simulink model "feedforward"  (R2017a)
settings: Solver=VariableStepAuto  StartTime=0.0  StopTime=20  RelTol=1e-3
libraries: simulink x1
settings Model: Creator=faari  LastModifiedBy=faari

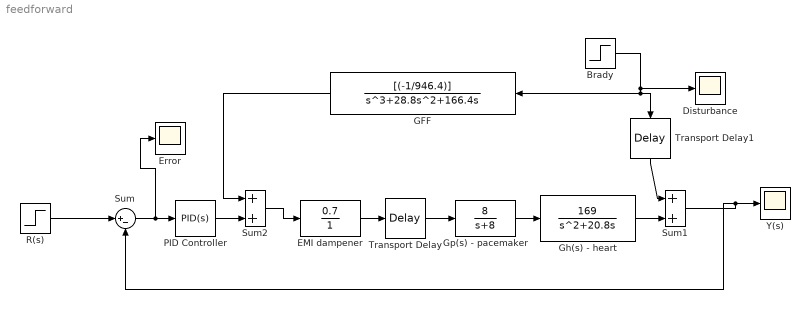
== system feedforward ==
  Brady : Step  Before=75  After=40  SampleTime=0
  Disturbance : Scope
  EMI dampener : TransferFcn  Numerator=[0.7]  Denominator=[1]
  Error : Scope
  GFF : TransferFcn  Numerator=[(-1/946.4)]  Denominator=[1 28.8 166.4 0]
  Gh(s) - heart : TransferFcn  Numerator=[169]  Denominator=[1 20.8 0]
  Gp(s) - pacemaker : TransferFcn  Numerator=[8]  Denominator=[1 8]
  PID Controller : simulink/Continuous/PID Controller  Controller=PID  TimeDomain=Continuous-time  SampleTime=-1  IntegratorMethod=Forward Euler  FilterMethod=Forward Euler  Form=Ideal  UseFilter=on  ControllerParametersSource=internal  P=0.475508627243744  I=0.245844606423706  D=0.157247274855767  N=100  InitialConditionSource=internal  InitialConditionForIntegrator=0  InitialConditionForFilter=0  ExternalReset=none  LimitOutput=off  UpperSaturationLimit=inf  LowerSaturationLimit=-inf  LinearizeAsGain=on  AntiWindupMode=none  Kb=1  TrackingMode=off  Kt=1  PParamMin=[]  PParamMax=[]  IParamMin=[]  IParamMax=[]  DParamMin=[]  DParamMax=[]  NParamMin=[]  NParamMax=[]  KbParamMin=[]  KbParamMax=[]  KtParamMin=[]  KtParamMax=[]  POutMin=[]  POutMax=[]  IOutMin=[]  IOutMax=[]  DOutMin=[]  DOutMax=[]  NOutMin=[]  NOutMax=[]  KbOutMin=[]  KbOutMax=[]  KtOutMin=[]  KtOutMax=[]  IntegratorOutMin=[]  IntegratorOutMax=[]  FilterOutMin=[]  FilterOutMax=[]  SumOutMin=[]  SumOutMax=[]  SumI1OutMin=[]  SumI1OutMax=[]  SumI2OutMin=[]  SumI2OutMax=[]  SumI3OutMin=[]  SumI3OutMax=[]  SumDOutMin=[]  SumDOutMax=[]  SaturationOutMin=[]  SaturationOutMax=[]  IntegratorContinuousStateAttributes=''  IntegratorStateMustResolveToSignalObject=off  IntegratorRTWStateStorageClass=Auto  FilterContinuousStateAttributes=''  FilterStateMustResolveToSignalObject=off  FilterRTWStateStorageClass=Auto  DifferentiatorICPrevScaledInput=0  DifferentiatorOutMin=[]  DifferentiatorOutMax=[]  InitialConditionSetting=State (most efficient)
  R(s) : Step  Time=0  After=75  SampleTime=0
  Sum : Sum  Inputs=|+-
  Sum1 : Sum  Inputs=+|+
  Sum2 : Sum  Inputs=+|+
  Transport Delay : TransportDelay  DelayTime=0.145
  Transport Delay1 : TransportDelay  DelayTime=0.145
  Y(s) : Scope
  wires:
  Sum/1 -> Error/1, PID Controller/1
  Gp(s) - pacemaker/1 -> Gh(s) - heart/1
  R(s)/1 -> Sum/1
  Gh(s) - heart/1 -> Sum1/2
  Sum1/1 -> Sum/2, Y(s)/1
  Transport Delay/1 -> Gp(s) - pacemaker/1
  EMI dampener/1 -> Transport Delay/1
  PID Controller/1 -> Sum2/2
  Brady/1 -> Disturbance/1, GFF/1, Transport Delay1/1
  Transport Delay1/1 -> Sum1/1
  GFF/1 -> Sum2/1
  Sum2/1 -> EMI dampener/1
